simulink model "controller1"  (R2022a)
settings: Solver=VariableStepAuto  StartTime=0.0  StopTime=10.0  RelTol=1e-3
undefined symbols (not defined in the file or in its folder): quant
settings Model: Creator=lixinru  LastModifiedBy=theod
settings SolverCC: AlgebraicLoopSolver=TrustRegion
settings DataIOCC: ReturnWorkspaceOutputs=off
settings DebuggingCC: UnconnectedInputMsg=warning  UnconnectedOutputMsg=warning  UnconnectedLineMsg=warning  SFMachineParentedDataDiag=warning  ArithmeticOperatorsInVariantConditions=warning
settings SFSimCC: SimUseLocalCustomCode=off  CustomCodeUndefinedFunction=UseInterfaceOnly
settings RTWCC: RTWUseLocalCustomCode=off

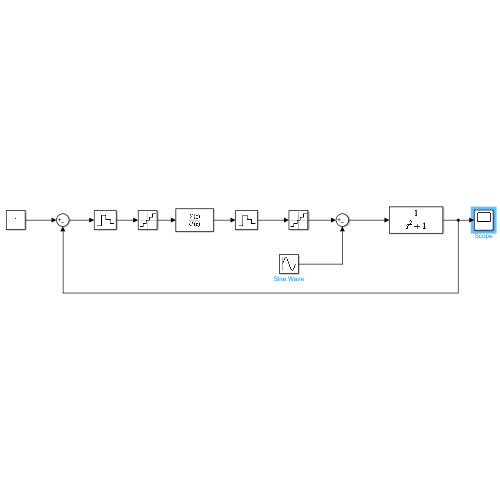
[thumbnail: Simulink's stored preview of the top-level diagram]
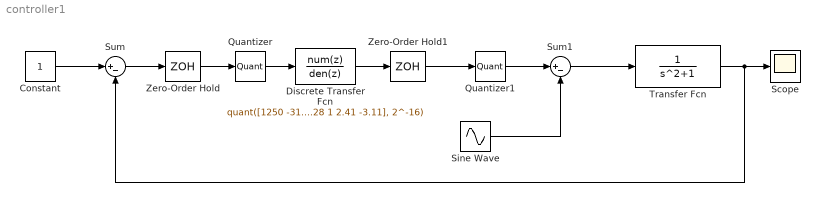
== system controller1 ==
  Constant : Constant
  Discrete Transfer Fcn : DiscreteTransferFcn  Numerator=quant([1250 -3150 3720 -2340 623], 2^-16)  Denominator=quant([1 1.99 -3.28 1 2.41 -3.11], 2^-16)
  Quantizer : Quantizer  QuantizationInterval=0.01
  Quantizer1 : Quantizer  QuantizationInterval=0.01
  Scope : Scope
  Sine Wave : Sin  Frequency=10  SampleTime=0
  Sum : Sum  Inputs=|+-
  Sum1 : Sum  Inputs=|+-
  Transfer Fcn : TransferFcn  Denominator=[1 0 1]
  Zero-Order Hold : ZeroOrderHold  SampleTime=0.1
  Zero-Order Hold1 : ZeroOrderHold  SampleTime=-1
  wires:
  Discrete Transfer Fcn/1 -> Zero-Order Hold1/1
  Zero-Order Hold/1 -> Quantizer/1
  Quantizer/1 -> Discrete Transfer Fcn/1
  Zero-Order Hold1/1 -> Quantizer1/1
  Constant/1 -> Sum/1
  Sum/1 -> Zero-Order Hold/1
  Transfer Fcn/1 -> Sum/2, Scope/1
  Quantizer1/1 -> Sum1/1
  Sum1/1 -> Transfer Fcn/1
  Sine Wave/1 -> Sum1/2
